simulink model "regulator"  (R2016b)
settings: Solver=ode14x  StartTime=0.0  StopTime=5  FixedStep=0.008  RelTol=1e-6  EnableMultiTasking=on
undefined symbols (not defined in the file): Kd, T2, w2, w3
libraries: simulink x1
settings Model: Creator=senserlex  LastModifiedBy=senserlex
settings SolverCC: InsertRTBMode=Always
settings DataIOCC: LimitDataPoints=on  SaveOutput=off  SaveTime=off
settings OptimizationCC: BlockReduction=off  BooleanDataType=off  LifeSpan=inf
settings DebuggingCC: SaveWithParameterizedLinksMsg=none  UnderspecifiedInitializationDetection=Classic  MergeDetectMultiDrivingBlocksExec=none  SignalResolutionControl=TryResolveAllWithWarning  AllowSymbolicDim=off  SFUnexpectedBacktrackingDiag=warning  SFNoUnconditionalDefaultTransitionDiag=warning  SFExecutionAtInitializationDiag=none
settings HardwareCC: TargetUnknown=on
settings GRTTargetCC: TargetLangStandard=C89/C90 (ANSI)  GeneratePreprocessorConditionals=Disable all

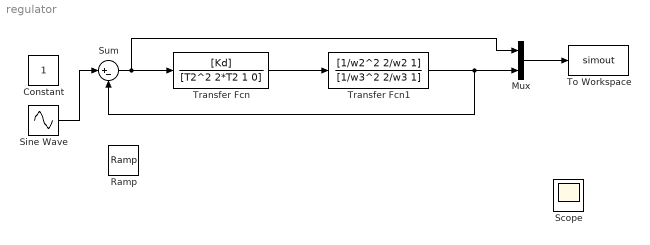
== system regulator ==
  Constant : Constant
  Mux : Mux  Inputs=2
  Ramp : simulink/Sources/Ramp  slope=5  start=0  X0=0
  Scope : Scope
  Sine Wave : Sin  Amplitude=0.8  Frequency=3  SampleTime=0
  Sum : Sum  Inputs=|+-
  To Workspace : ToWorkspace  VariableName=simout  SaveFormat=Timeseries  SampleTime=-1
  Transfer Fcn : TransferFcn  Numerator=[Kd]  Denominator=[T2^2 2*T2 1 0]
  Transfer Fcn1 : TransferFcn  Numerator=[1/w2^2 2/w2 1]  Denominator=[1/w3^2 2/w3 1]
  wires:
  Sum/1 -> Transfer Fcn/1, Mux/1
  Transfer Fcn1/1 -> Sum/2, Mux/2
  Transfer Fcn/1 -> Transfer Fcn1/1
  Mux/1 -> To Workspace/1
  Sine Wave/1 -> Sum/1
